simulink model "TSCLAB_ModelPV_15"  (R2020a)
settings: Solver=VariableStepAuto  StartTime=0.0  StopTime=200  RelTol=1e-3
undefined symbols (not defined in the file or in its folder): serial
libraries: instrumentlib x3
settings Model: Creator=vasanza  LastModifiedBy=Familia Zúñiga Vega
settings DebuggingCC: ArithmeticOperatorsInVariantConditions=warning
settings SFSimCC: CustomCodeUndefinedFunction=UseInterfaceOnly

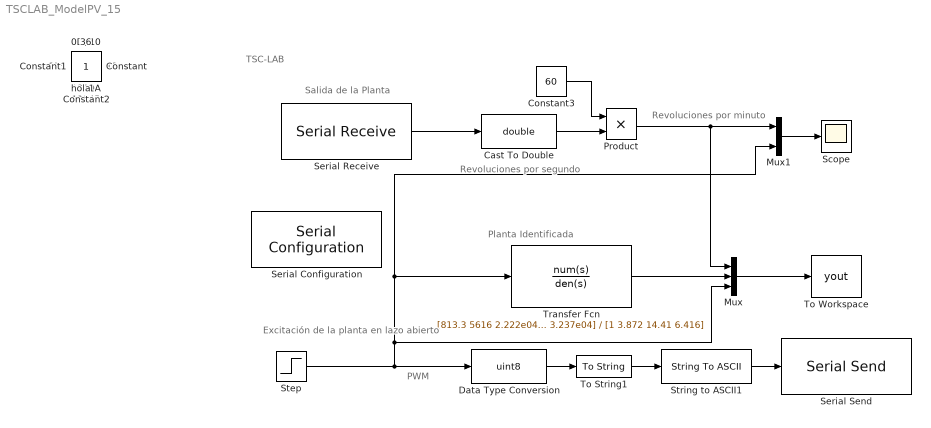
== system TSCLAB_ModelPV_15 ==
  note: PWM
  note: Excitación de la planta en lazo abierto
  note: Planta Identificada
  note: Revoluciones por minuto
  note: Revoluciones por segundo
  note: Salida de la Planta
  note: TSC-LAB
  Cast To Double : DataTypeConversion  OutDataTypeStr=double
  Constant3 : Constant  Value=60
  Data Type Conversion : DataTypeConversion  OutDataTypeStr=uint8
  Mux : Mux  Inputs=3
  Mux1 : Mux  Inputs=2
  Product : Product
  Scope : Scope
  Serial Configuration : instrumentlib/Serial Configuration  Priority=-200000  ComPortMenu=COM24  ComPort=COM31  ObjConstructor=serial('COM31');  BaudRate=115200  DataBits=8  Parity=none  FlowControl=none  Timeout=10  ByteOrder=LittleEndian
  Serial Receive : instrumentlib/Serial Receive  ComPortMenu=COM30  ComPort=COM31  ObjConstructor=serial('COM31');  Terminator=<none>  DataSize=[1 1]  DataType=uint8  EnableBlockingMode=on  ActionDataUnavailable=Output last received value  CustomValue=0  SampleTime=0.249
  Serial Send : instrumentlib/Serial Send  ComPortMenu=COM30  ComPort=COM31  ObjConstructor=serial('COM31');  Terminator=<none>  EnableBlockingMode=on
  Step : Step  After=255  SampleTime=0.999
  String to ASCII1 : StringToASCII
  To String1 : ToString
  To Workspace : ToWorkspace  VariableName=yout  SampleTime=-1
      settings: Save2DSignal=2-D array (concatenate along first dimension)
  Transfer Fcn : TransferFcn  Numerator=[813.3 5616 2.222e04 3.237e04]  Denominator=[1 3.872 14.41 6.416]
  $ : Constant  IOType=siggen  Value=36
  , : Constant  IOType=siggen  Value=44
  {0,10,255,311,12345} (5 alike) : Constant  IOType=siggen
  0A : Constant  IOType=siggen  Value=10
  0D : Constant  IOType=siggen  Value=13
  13 : Constant  IOType=siggen  Value=13
  36 : Constant  IOType=siggen  Value=36
  Constant : Constant  IOType=siggen
  Constant1 : Constant  IOType=siggen
  Constant2 : Constant  IOType=siggen
  hola : Constant  IOType=siggen
  wires:
  Mux/1 -> To Workspace/1
  Transfer Fcn/1 -> Mux/2
  Data Type Conversion/1 -> To String1/1
  Serial Receive/1 -> Cast To Double/1
  Mux1/1 -> Scope/1
  Step/1 -> Data Type Conversion/1, Mux/3, Transfer Fcn/1, Mux1/2
  Cast To Double/1 -> Product/2
  Constant3/1 -> Product/1
  Product/1 -> Mux/1, Mux1/1
  String to ASCII1/1 -> Serial Send/1
  To String1/1 -> String to ASCII1/1
